simulink model "Differential_Jacobian_mapping_Model"  (R2016a)
settings: Solver=FixedStepAuto  SolverMode=SingleTasking  StartTime=0  StopTime=2  FixedStep=0.04  RelTol=1e-3
undefined symbols (not defined in the file): display, Z
libraries: sm_lib x176, nesl_utility x21, simulink x10
(part 2 of 2)

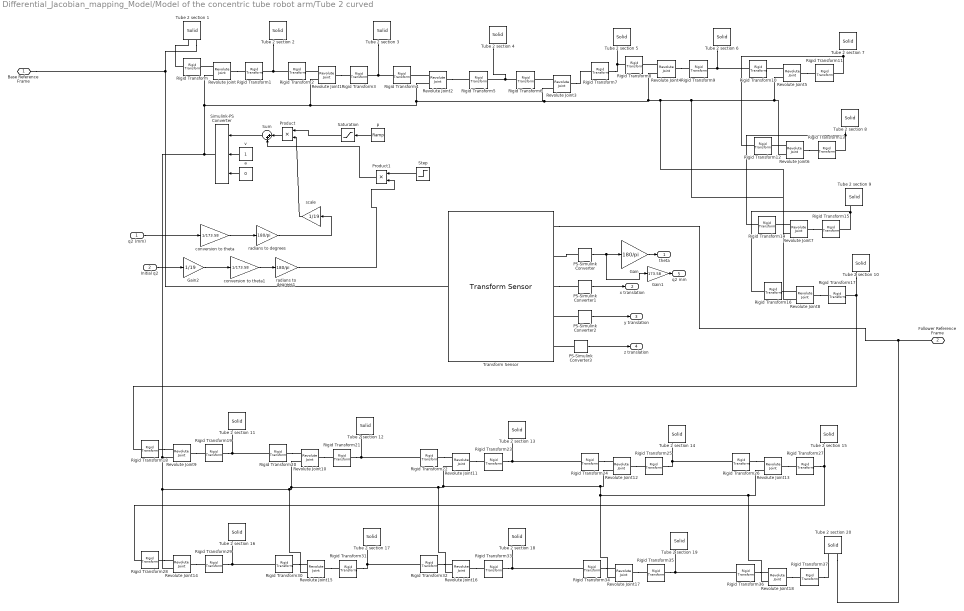
== system Differential_Jacobian_mapping_Model/Model of the concentric tube robot arm/Tube 2 curved ==
  q2 (mm) : Inport
  Initial q2 : Inport  Port=2
  Gain : Gain  Gain=180/pi
  Gain1 : Gain  Gain=173.58
  Gain2 : Gain  Gain=1/19
  PS-Simulink Converter{,1..3} (4 alike) : nesl_utility/PS-Simulink Converter  PhysicalDomain=network_engine_domain  SubClassName=ps_output  LeftPortType=input  RightPortType=output  PseudoPeriodic=off  Frequencies=[]  Unit=1  AffineConversion=off
  Product : Product
  Product1 : Product
  Revolute Joint{,1..18} (19 alike) : sm_lib/Joints/Revolute Joint  SenseConstraintForce=off  SenseConstraintForceX=off  SenseConstraintForceY=off  SenseConstraintForceZ=off  SenseConstraintTorque=off  SenseConstraintTorqueX=off  SenseConstraintTorqueY=off  SenseConstraintTorqueZ=off  SenseTotalForce=off  SenseTotalForceX=off  SenseTotalForceY=off  SenseTotalForceZ=off  SenseTotalTorque=off  SenseTotalTorqueX=off  SenseTotalTorqueY=off  SenseTotalTorqueZ=off  CompositeWrenchDir=FollowerOnBase  CompositeWrenchFrame=BaseFrame  EquilibriumPosition=0  EquilibriumPositionUnits=deg  SpringStiffness=0  SpringStiffnessUnits=N*m/deg  DampingCoefficient=0  DampingCoefficientUnits=N*m/(deg/s)  TorqueActuationMode=ComputedTorque  MotionActuationMode=InputMotion  SensePosition=off  SenseVelocity=off  SenseAcceleration=off  SenseTorqueForce=off  PositionTargetSpecify=off  PositionTargetPriority=High  PositionTargetValue=0  PositionTargetValueUnits=deg  VelocityTargetSpecify=off  VelocityTargetPriority=High  VelocityTargetValue=0  VelocityTargetValueUnits=deg/s
  Rigid Transform{,2,4,6,8,10,12,14,16,18,20,22,24,26,28,30,32,34,36} (19 alike) : sm_lib/Frames and Transforms/Rigid Transform  TranslationMethod=StandardAxis  TranslationLengthUnit=mm  TranslationStandardAxis=-X  TranslationStandardOffset=173.58  TranslationCartesianOffset=[0 0 0]  TranslationROffset=0  TranslationROffsetUnits=m  TranslationZOffset=0  TranslationZOffsetUnits=m  TranslationThetaOffset=0  TranslationThetaOffsetUnits=deg  RotationMethod=StandardAxis  RotationAngleUnits=deg  RotationStandardAxis=+X  RotationAngle=90  RotationArbitraryAxis=[0 0 1]  FollAlignAxisA=+X  BaseAlignAxisA=+Y  FollAlignAxisB=+Y  BaseAlignAxisB=+Z  RotationSequenceAxes=FollowerAxes  RotationSequence=XYX  RotationSequenceAngles=[0 0 0]  RotationSequenceAnglesUnits=deg  RotationMatrix=[1 0 0; 0 1 0; 0 0 1]
  Rigid Transform{1,3,5,7,9,11,13,15,17,19,21,23,25,27,29,31,33,35,37} (19 alike) : sm_lib/Frames and Transforms/Rigid Transform  TranslationMethod=StandardAxis  TranslationLengthUnit=mm  TranslationStandardAxis=+X  TranslationStandardOffset=173.58  TranslationCartesianOffset=[0 0 0]  TranslationROffset=0  TranslationROffsetUnits=m  TranslationZOffset=0  TranslationZOffsetUnits=m  TranslationThetaOffset=0  TranslationThetaOffsetUnits=deg  RotationMethod=StandardAxis  RotationAngleUnits=deg  RotationStandardAxis=-X  RotationAngle=90  RotationArbitraryAxis=[0 0 1]  FollAlignAxisA=+X  BaseAlignAxisA=+Y  FollAlignAxisB=+Y  BaseAlignAxisB=+Z  RotationSequenceAxes=FollowerAxes  RotationSequence=XYX  RotationSequenceAngles=[0 0 0]  RotationSequenceAnglesUnits=deg  RotationMatrix=[1 0 0; 0 1 0; 0 0 1]
  Saturation : Saturate  UpperLimit=1  LowerLimit=0
  Simulink-PS Converter : nesl_utility/Simulink-PS Converter  PhysicalDomain=network_engine_domain  SubClassName=ps_input  LeftPortType=input  RightPortType=output  PseudoPeriodic=off  Frequencies=[]  NoiseDistribution=none  NoiseParameters=[]  Unit=deg  AffineConversion=off  InputFiltering=derivs  SimscapeFilterOrder=1  InputFilterTimeConstant=0.001  UdotUserProvided=2
  Step : Step  Time=0  SampleTime=0
  Sum : Sum  Inputs=|++
  Transform Sensor : sm_lib/Frames and Transforms/Transform Sensor  MeasurementFrame=Base  SenseAngle=on  SenseAxis=off  SenseAngle1=off  SenseAngle2=off  SenseAngle3=off  SenseQ=off  SenseR=off  SenseOmegaX=off  SenseOmegaY=off  SenseOmegaZ=off  SenseOmega1=off  SenseOmega2=off  SenseOmega3=off  SenseQDot=off  SenseRDot=off  SenseAlphaX=off  SenseAlphaY=off  SenseAlphaZ=off  SenseAlpha1=off  SenseAlpha2=off  SenseAlpha3=off  SenseQDDot=off  SenseRDDot=off  SenseX=on  SenseY=on  SenseZ=on  SenseRad=off  SenseAzim=off  SenseDist=off  SenseInc=off  SenseXDot=off  SenseYDot=off  SenseZDot=off  SenseRadDot=off  SenseAzimDot=off  SenseDistDot=off  SenseIncDot=off  SenseXDDot=off  SenseYDDot=off  SenseZDDot=off  SenseRadDDot=off  SenseAzimDDot=off  SenseDistDDot=off  SenseIncDDot=off
  Tube 2 section {1..20} (20 alike) : sm_lib/Body Elements/Solid  InertiaType=CalculateFromGeometry  Mass=1  MassUnits=kg  CenterOfMass=[0 0 0]  CenterOfMassUnits=m  MomentsOfInertia=[1 1 1]  MomentsOfInertiaUnits=kg*m^2  ProductsOfInertia=[0 0 0]  ProductsOfInertiaUnits=kg*m^2  DensityBased=on  Density=1000  DensityUnits=kg/(m^3)  DoExposeReferenceFrame=on  SerializedFrames=<Frames><Frame><Id>Frame1</Id><Value><Name>F1</Name><Origin><Source>GeometricFeature</Source><FeatureName>back surface</FeatureName></Origin><PrimaryAxis><DefinedDirection>-Z</DefinedDirection><Source>GeometricFeature</Source><SourceDirection>+Z</SourceDirection><FeatureName>back surface</FeatureName></PrimaryAxis><SecondaryAxis><DefinedDirection>+X</DefinedDirection><Source>ReferenceFrame</Source><SourceDirection>+X</SourceDirection><FeatureName></FeatureName></SecondaryAxis></Value></Frame><Frame><Id>Frame2</Id><Value><Name>F2</Name><Origin><Source>GeometricFeature</Source><FeatureName>front surface</FeatureName></Origin><PrimaryAxis><DefinedDirection>+Z</DefinedDirection><Source>GeometricFeature</Source><SourceDirection>+Z</SourceDirection><FeatureName>front surface</FeatureName></PrimaryAxis><SecondaryAxis><DefinedDirection>+X</DefinedDirection><Source>ReferenceFrame</Source><SourceDirection>+X</SourceDirection><FeatureName></FeatureName></SecondaryAxis></Value></Frame></Frames>  GraphicType=FromGeometry  MarkerShape=Sphere  MarkerSize=10  GraphicVisPropType=SimpleVisualProperties  GraphicDiffuseColor=[0.5 0.5 0.5]  GraphicSpecularColor=[0.5 0.5 0.5 1.0]  GraphicAmbientColor=[0.15 0.15 0.15 1.0]  GraphicEmissiveColor=[0.0 0.0 0.0 1.0]  GraphicShininess=75  GraphicOpacity=1.0  GeometryShape=GeneralSolidOfRevolution  RectangleSize=[1 1]  RectangleSizeUnits=m  BrickDimensions=[1 1 1]  BrickDimensionUnits=m  CylinderRadius=3  CylinderRadiusUnits=mm  CylinderLength=q1  CylinderLengthUnits=mm  SphereRadius=1  SphereRadiusUnits=m  EllipsoidRadii=[1 1 1]  EllipsoidRadiiUnits=m  ExtrusionCrossSection=[1 1; -1 1; -1 -1; 1 -1]  ExtrusionCrossSectionUnits=m  ExtrusionLength=1  ExtrusionLengthUnits=m  PolygonNumSides=3  PolygonOuterRadius=1  PolygonOuterRadiusUnits=m  ExtGeomFileType=STEP  ExtGeomFileUnits=m  RevolutionCrossSection=Cross_section_tube2  RevolutionCrossSectionUnits=mm  RevolutionExtent=Custom  RevolutionAngle=5  RevolutionAngleUnits=deg
  a : Constant  Value=0
  conversion to theta : Gain  Gain=1/173.58
  conversion to theta1 : Gain  Gain=1/173.58
  p : simulink/Sources/Ramp  slope=1  start=0  X0=0
  radians to degrees : Gain  Gain=180/pi
  radians to degrees1 : Gain  Gain=180/pi
  scale : Gain  Gain=1/19
  v : Constant
  Base Reference Frame : PMIOPort  Port=1  Side=Left
  Follower Reference Frame : PMIOPort  Port=2  Side=Right
  theta : Outport
  x translation : Outport  Port=2
  y translation : Outport  Port=3
  z translation : Outport  Port=4
  q2 mm : Outport  Port=5
  wires:
  a/1 -> Simulink-PS Converter/3
  v/1 -> Simulink-PS Converter/2
  p/1 -> Saturation/1
  PS-Simulink Converter/1 -> Gain1/1, Gain/1
  Gain/1 -> theta/1
  Saturation/1 -> Product/1
  conversion to theta/1 -> radians to degrees/1
  PS-Simulink Converter1/1 -> x translation/1
  PS-Simulink Converter2/1 -> y translation/1
  PS-Simulink Converter3/1 -> z translation/1
  q2 (mm)/1 -> conversion to theta/1
  Product1/1 -> Sum/2
  Step/1 -> Product1/1
  radians to degrees1/1 -> Product1/2
  conversion to theta1/1 -> radians to degrees1/1
  radians to degrees/1 -> scale/1
  Initial q2/1 -> Gain2/1
  Gain2/1 -> conversion to theta1/1
  Gain1/1 -> q2 mm/1
  scale/1 -> Product/2
  Product/1 -> Sum/1
  Sum/1 -> Simulink-PS Converter/1
  connections:
  Rigid Transform/LConn1 -- Tube 2 section 1/LConn1
  Rigid Transform1/RConn1 -- Tube 2 section 2/LConn1 -- Rigid Transform2/LConn1
  Revolute Joint/LConn2 -- Revolute Joint8/LConn2 -- Revolute Joint7/LConn2 -- Revolute Joint6/LConn2 -- Revolute Joint5/LConn2 -- Revolute Joint4/LConn2 -- Revolute Joint3/LConn2 -- Revolute Joint2/LConn2 -- Revolute Joint1/LConn2 -- Revolute Joint18/LConn2 -- Revolute Joint13/LConn2 -- Revolute Joint17/LConn2 -- Revolute Joint12/LConn2 -- Revolute Joint11/LConn2 -- Revolute Joint16/LConn2 -- Revolute Joint10/LConn2 -- Revolute Joint15/LConn2 -- Revolute Joint14/LConn2 -- Revolute Joint9/LConn2 -- Simulink-PS Converter/RConn1
  Rigid Transform3/RConn1 -- Tube 2 section 3/LConn1 -- Rigid Transform4/LConn1
  Rigid Transform6/LConn1 -- Tube 2 section 4/LConn1 -- Rigid Transform5/RConn1
  Tube 2 section 5/LConn1 -- Rigid Transform7/RConn1 -- Rigid Transform8/LConn1
  Rigid Transform10/LConn1 -- Tube 2 section 6/LConn1 -- Rigid Transform9/RConn1
  Rigid Transform12/LConn1 -- Tube 2 section 7/LConn1 -- Rigid Transform11/RConn1
  Rigid Transform13/RConn1 -- Tube 2 section 8/LConn1 -- Rigid Transform14/LConn1
  Rigid Transform16/LConn1 -- Tube 2 section 9/LConn1 -- Rigid Transform15/RConn1
  Transform Sensor/RConn1 -- Tube 2 section 20/LConn2 -- Follower Reference Frame/RConn1
  Revolute Joint8/RConn1 -- Rigid Transform17/LConn1
  Revolute Joint1/RConn1 -- Rigid Transform3/LConn1
  Revolute Joint8/LConn1 -- Rigid Transform16/RConn1
  Revolute Joint2/LConn1 -- Rigid Transform4/RConn1
  Tube 2 section 10/LConn1 -- Rigid Transform18/LConn1 -- Rigid Transform17/RConn1
  Revolute Joint7/RConn1 -- Rigid Transform15/LConn1
  Revolute Joint7/LConn1 -- Rigid Transform14/RConn1
  Tube 2 section 1/LConn2 -- Base Reference Frame/RConn1 -- Transform Sensor/LConn1
  Revolute Joint3/RConn1 -- Rigid Transform7/LConn1
  PS-Simulink Converter/LConn1 -- Transform Sensor/RConn2
  Revolute Joint5/RConn1 -- Rigid Transform11/LConn1
  Revolute Joint4/RConn1 -- Rigid Transform9/LConn1
  Revolute Joint/RConn1 -- Rigid Transform1/LConn1
  Revolute Joint/LConn1 -- Rigid Transform/RConn1
  Revolute Joint1/LConn1 -- Rigid Transform2/RConn1
  Revolute Joint2/RConn1 -- Rigid Transform5/LConn1
  Revolute Joint3/LConn1 -- Rigid Transform6/RConn1
  Revolute Joint6/RConn1 -- Rigid Transform13/LConn1
  Revolute Joint4/LConn1 -- Rigid Transform8/RConn1
  Revolute Joint5/LConn1 -- Rigid Transform10/RConn1
  Revolute Joint6/LConn1 -- Rigid Transform12/RConn1
  PS-Simulink Converter3/LConn1 -- Transform Sensor/RConn5
  PS-Simulink Converter2/LConn1 -- Transform Sensor/RConn4
  Transform Sensor/RConn3 -- PS-Simulink Converter1/LConn1
  Rigid Transform18/RConn1 -- Revolute Joint9/LConn1
  Revolute Joint9/RConn1 -- Rigid Transform19/LConn1
  Rigid Transform19/RConn1 -- Rigid Transform20/LConn1 -- Tube 2 section 11/LConn1
  Rigid Transform20/RConn1 -- Revolute Joint10/LConn1
  Revolute Joint10/RConn1 -- Rigid Transform21/LConn1
  Rigid Transform21/RConn1 -- Tube 2 section 12/LConn1 -- Rigid Transform22/LConn1
  Rigid Transform22/RConn1 -- Revolute Joint11/LConn1
  Revolute Joint11/RConn1 -- Rigid Transform23/LConn1
  Rigid Transform23/RConn1 -- Rigid Transform24/LConn1 -- Tube 2 section 13/LConn1
  Rigid Transform24/RConn1 -- Revolute Joint12/LConn1
  Revolute Joint12/RConn1 -- Rigid Transform25/LConn1
  Rigid Transform25/RConn1 -- Rigid Transform26/LConn1 -- Tube 2 section 14/LConn1
  Rigid Transform26/RConn1 -- Revolute Joint13/LConn1
  Revolute Joint13/RConn1 -- Rigid Transform27/LConn1
  Rigid Transform27/RConn1 -- Rigid Transform28/LConn1 -- Tube 2 section 15/LConn1
  Rigid Transform28/RConn1 -- Revolute Joint14/LConn1
  Revolute Joint14/RConn1 -- Rigid Transform29/LConn1
  Rigid Transform29/RConn1 -- Rigid Transform30/LConn1 -- Tube 2 section 16/LConn1
  Rigid Transform30/RConn1 -- Revolute Joint15/LConn1
  Revolute Joint15/RConn1 -- Rigid Transform31/LConn1
  Rigid Transform31/RConn1 -- Rigid Transform32/LConn1 -- Tube 2 section 17/LConn1
  Rigid Transform32/RConn1 -- Revolute Joint16/LConn1
  Revolute Joint16/RConn1 -- Rigid Transform33/LConn1
  Rigid Transform33/RConn1 -- Rigid Transform34/LConn1 -- Tube 2 section 18/LConn1
  Rigid Transform34/RConn1 -- Revolute Joint17/LConn1
  Revolute Joint17/RConn1 -- Rigid Transform35/LConn1
  Rigid Transform35/RConn1 -- Rigid Transform36/LConn1 -- Tube 2 section 19/LConn1
  Rigid Transform36/RConn1 -- Revolute Joint18/LConn1
  Revolute Joint18/RConn1 -- Rigid Transform37/LConn1
  Rigid Transform37/RConn1 -- Tube 2 section 20/LConn1

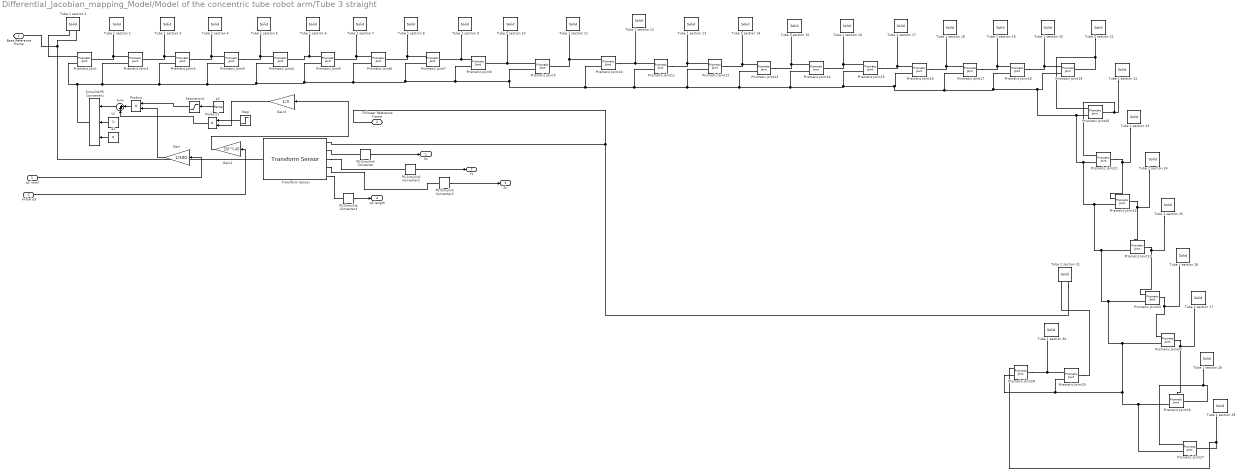
== system Differential_Jacobian_mapping_Model/Model of the concentric tube robot arm/Tube 3 straight ==
  q3 (mm) : Inport
  Initial q3 : Inport  Port=2
  Gain : Gain  Gain=1/300
  Gain2 : Gain  Gain=10^(-4)
  Gain3 : Gain  Gain=1/3
  PS-Simulink Converter{,1..3} (4 alike) : nesl_utility/PS-Simulink Converter  PhysicalDomain=network_engine_domain  SubClassName=ps_output  LeftPortType=input  RightPortType=output  PseudoPeriodic=off  Frequencies=[]  Unit=1  AffineConversion=off
  Prismatic Joint{,1..29} (30 alike) : sm_lib/Joints/Prismatic Joint  SenseConstraintForce=off  SenseConstraintForceX=off  SenseConstraintForceY=off  SenseConstraintForceZ=off  SenseConstraintTorque=off  SenseConstraintTorqueX=off  SenseConstraintTorqueY=off  SenseConstraintTorqueZ=off  SenseTotalForce=off  SenseTotalForceX=off  SenseTotalForceY=off  SenseTotalForceZ=off  SenseTotalTorque=off  SenseTotalTorqueX=off  SenseTotalTorqueY=off  SenseTotalTorqueZ=off  CompositeWrenchDir=FollowerOnBase  CompositeWrenchFrame=BaseFrame  EquilibriumPosition=0  EquilibriumPositionUnits=m  SpringStiffness=0  SpringStiffnessUnits=N/m  DampingCoefficient=0  DampingCoefficientUnits=N/(m/s)  TorqueActuationMode=ComputedTorque  MotionActuationMode=InputMotion  SensePosition=off  SenseVelocity=off  SenseAcceleration=off  SenseTorqueForce=off  PositionTargetSpecify=off  PositionTargetPriority=High  PositionTargetValue=0  PositionTargetValueUnits=m  VelocityTargetSpecify=off  VelocityTargetPriority=High  VelocityTargetValue=0  VelocityTargetValueUnits=m/s
  Product : Product
  Product1 : Product
  Saturation1 : Saturate  UpperLimit=0.01  LowerLimit=0
  Simulink-PS Converter1 : nesl_utility/Simulink-PS Converter  PhysicalDomain=network_engine_domain  SubClassName=ps_input  LeftPortType=input  RightPortType=output  PseudoPeriodic=off  Frequencies=[]  NoiseDistribution=none  NoiseParameters=[]  Unit=m  AffineConversion=off  InputFiltering=derivs  SimscapeFilterOrder=1  InputFilterTimeConstant=0.001  UdotUserProvided=2
  Step : Step  Time=0  SampleTime=0
  Sum : Sum  Inputs=|++
  Transform Sensor : sm_lib/Frames and Transforms/Transform Sensor  MeasurementFrame=Base  SenseAngle=off  SenseAxis=off  SenseAngle1=off  SenseAngle2=off  SenseAngle3=off  SenseQ=off  SenseR=off  SenseOmegaX=off  SenseOmegaY=off  SenseOmegaZ=off  SenseOmega1=off  SenseOmega2=off  SenseOmega3=off  SenseQDot=off  SenseRDot=off  SenseAlphaX=off  SenseAlphaY=off  SenseAlphaZ=off  SenseAlpha1=off  SenseAlpha2=off  SenseAlpha3=off  SenseQDDot=off  SenseRDDot=off  SenseX=on  SenseY=on  SenseZ=on  SenseRad=off  SenseAzim=off  SenseDist=on  SenseInc=off  SenseXDot=off  SenseYDot=off  SenseZDot=off  SenseRadDot=off  SenseAzimDot=off  SenseDistDot=off  SenseIncDot=off  SenseXDDot=off  SenseYDDot=off  SenseZDDot=off  SenseRadDDot=off  SenseAzimDDot=off  SenseDistDDot=off  SenseIncDDot=off
  Tube 1 section {1..31} (31 alike) : sm_lib/Body Elements/Solid  InertiaType=CalculateFromGeometry  Mass=1  MassUnits=kg  CenterOfMass=[0 0 0]  CenterOfMassUnits=m  MomentsOfInertia=[1 1 1]  MomentsOfInertiaUnits=kg*m^2  ProductsOfInertia=[0 0 0]  ProductsOfInertiaUnits=kg*m^2  DensityBased=on  Density=0  DensityUnits=kg/(m^3)  DoExposeReferenceFrame=on  SerializedFrames=<Frames><Frame><Id>Frame1</Id><Value><Name>F1</Name><Origin><Source>GeometricFeature</Source><FeatureName>bottom surface</FeatureName></Origin><PrimaryAxis><DefinedDirection>+Z</DefinedDirection><Source>ReferenceFrame</Source><SourceDirection>+Z</SourceDirection><FeatureName></FeatureName></PrimaryAxis><SecondaryAxis><DefinedDirection>+X</DefinedDirection><Source>ReferenceFrame</Source><SourceDirection>+X</SourceDirection><FeatureName></FeatureName></SecondaryAxis></Value></Frame><Frame><Id>Frame2</Id><Value><Name>F2</Name><Origin><Source>GeometricFeature</Source><FeatureName>top surface</FeatureName></Origin><PrimaryAxis><DefinedDirection>+Z</DefinedDirection><Source>ReferenceFrame</Source><SourceDirection>+Z</SourceDirection><FeatureName></FeatureName></PrimaryAxis><SecondaryAxis><DefinedDirection>+X</DefinedDirection><Source>ReferenceFrame</Source><SourceDirection>+X</SourceDirection><FeatureName></FeatureName></SecondaryAxis></Value></Frame></Frames>  GraphicType=FromGeometry  MarkerShape=Sphere  MarkerSize=10  GraphicVisPropType=SimpleVisualProperties  GraphicDiffuseColor=[0.5 0.5 0.5]  GraphicSpecularColor=[0.5 0.5 0.5 1.0]  GraphicAmbientColor=[0.15 0.15 0.15 1.0]  GraphicEmissiveColor=[0.0 0.0 0.0 1.0]  GraphicShininess=75  GraphicOpacity=1.0  GeometryShape=Cylinder  RectangleSize=[1 1]  RectangleSizeUnits=m  BrickDimensions=[1 1 1]  BrickDimensionUnits=m  CylinderRadius=0.5  CylinderRadiusUnits=mm  CylinderLength=10  CylinderLengthUnits=mm  SphereRadius=1  SphereRadiusUnits=m  EllipsoidRadii=[1 1 1]  EllipsoidRadiiUnits=m  ExtrusionCrossSection=[1 1; -1 1; -1 -1; 1 -1]  ExtrusionCrossSectionUnits=m  ExtrusionLength=1  ExtrusionLengthUnits=m  PolygonNumSides=3  PolygonOuterRadius=1  PolygonOuterRadiusUnits=m  ExtGeomFileType=STEP  ExtGeomFileUnits=m  RevolutionCrossSection=[1 1; 1 -1; 2 -1; 2 1]  RevolutionCrossSectionUnits=m  RevolutionExtent=Full  RevolutionAngle=180  RevolutionAngleUnits=deg
  a1 : Constant  Value=0
  p1 : simulink/Sources/Ramp  slope=0.01  start=0  X0=0
  v1 : Constant
  Base Reference Frame : PMIOPort  Port=1  Side=Left
  Follower Reference Frame : PMIOPort  Port=2  Side=Right
  Xc : Outport
  Yc : Outport  Port=2
  Zc : Outport  Port=3
  q3 length : Outport  Port=4
  wires:
  a1/1 -> Simulink-PS Converter1/3
  v1/1 -> Simulink-PS Converter1/2
  p1/1 -> Saturation1/1
  PS-Simulink Converter/1 -> Xc/1
  PS-Simulink Converter1/1 -> Yc/1
  PS-Simulink Converter2/1 -> Zc/1
  PS-Simulink Converter3/1 -> q3 length/1
  q3 (mm)/1 -> Gain/1
  Step/1 -> Product1/1
  Product1/1 -> Sum/2
  Initial q3/1 -> Gain2/1
  Gain2/1 -> Gain3/1
  Gain3/1 -> Product1/2
  Saturation1/1 -> Product/1
  Product/1 -> Sum/1
  Gain/1 -> Product/2
  Sum/1 -> Simulink-PS Converter1/1
  connections:
  Simulink-PS Converter1/RConn1 -- Prismatic Joint/LConn2 -- Prismatic Joint29/LConn2 -- Prismatic Joint28/LConn2 -- Prismatic Joint27/LConn2 -- Prismatic Joint26/LConn2 -- Prismatic Joint25/LConn2 -- Prismatic Joint24/LConn2 -- Prismatic Joint23/LConn2 -- Prismatic Joint22/LConn2 -- Prismatic Joint21/LConn2 -- Prismatic Joint20/LConn2 -- Prismatic Joint19/LConn2 -- Prismatic Joint18/LConn2 -- Prismatic Joint17/LConn2 -- Prismatic Joint16/LConn2 -- Prismatic Joint15/LConn2 -- Prismatic Joint14/LConn2 -- Prismatic Joint13/LConn2 -- Prismatic Joint12/LConn2 -- Prismatic Joint11/LConn2 -- Prismatic Joint10/LConn2 -- Prismatic Joint9/LConn2 -- Prismatic Joint8/LConn2 -- Prismatic Joint7/LConn2 -- Prismatic Joint6/LConn2 -- Prismatic Joint5/LConn2 -- Prismatic Joint4/LConn2 -- Prismatic Joint3/LConn2 -- Prismatic Joint2/LConn2 -- Prismatic Joint1/LConn2
  Tube 1 section 1/LConn1 -- Prismatic Joint/LConn1
  Prismatic Joint1/LConn1 -- Prismatic Joint/RConn1 -- Tube 1 section 2/LConn1
  Prismatic Joint2/LConn1 -- Prismatic Joint1/RConn1 -- Tube 1 section 3/LConn1
  Prismatic Joint3/LConn1 -- Tube 1 section 4/LConn1 -- Prismatic Joint2/RConn1
  Prismatic Joint4/LConn1 -- Tube 1 section 5/LConn1 -- Prismatic Joint3/RConn1
  Prismatic Joint4/RConn1 -- Tube 1 section 6/LConn1 -- Prismatic Joint5/LConn1
  Prismatic Joint6/LConn1 -- Prismatic Joint5/RConn1 -- Tube 1 section 7/LConn1
  Prismatic Joint7/LConn1 -- Prismatic Joint6/RConn1 -- Tube 1 section 8/LConn1
  Prismatic Joint8/LConn1 -- Prismatic Joint7/RConn1 -- Tube 1 section 9/LConn1
  Prismatic Joint9/LConn1 -- Tube 1 section 10/LConn1 -- Prismatic Joint8/RConn1
  Prismatic Joint9/RConn1 -- Prismatic Joint10/LConn1 -- Tube 1 section 11/LConn1
  Transform Sensor/LConn1 -- Base Reference Frame/RConn1 -- Tube 1 section 1/LConn2
  Follower Reference Frame/RConn1 -- Tube 1 section 31/LConn2 -- Transform Sensor/RConn1
  PS-Simulink Converter/LConn1 -- Transform Sensor/RConn2
  Transform Sensor/RConn3 -- PS-Simulink Converter1/LConn1
  Transform Sensor/RConn4 -- PS-Simulink Converter2/LConn1
  Prismatic Joint10/RConn1 -- Tube 1 section 12/LConn1 -- Prismatic Joint11/LConn1
  Prismatic Joint11/RConn1 -- Prismatic Joint12/LConn1 -- Tube 1 section 13/LConn1
  Prismatic Joint12/RConn1 -- Prismatic Joint13/LConn1 -- Tube 1 section 14/LConn1
  Prismatic Joint13/RConn1 -- Prismatic Joint14/LConn1 -- Tube 1 section 15/LConn1
  Prismatic Joint14/RConn1 -- Prismatic Joint15/LConn1 -- Tube 1 section 16/LConn1
  Prismatic Joint15/RConn1 -- Prismatic Joint16/LConn1 -- Tube 1 section 17/LConn1
  Prismatic Joint16/RConn1 -- Prismatic Joint17/LConn1 -- Tube 1 section 18/LConn1
  Prismatic Joint17/RConn1 -- Prismatic Joint18/LConn1 -- Tube 1 section 19/LConn1
  Prismatic Joint18/RConn1 -- Prismatic Joint19/LConn1 -- Tube 1 section 20/LConn1
  Tube 1 section 21/LConn1 -- Prismatic Joint20/LConn1 -- Prismatic Joint19/RConn1
  Tube 1 section 22/LConn1 -- Prismatic Joint21/LConn1 -- Prismatic Joint20/RConn1
  Prismatic Joint21/RConn1 -- Tube 1 section 23/LConn1 -- Prismatic Joint22/LConn1
  Prismatic Joint22/RConn1 -- Tube 1 section 24/LConn1 -- Prismatic Joint23/LConn1
  Prismatic Joint23/RConn1 -- Tube 1 section 25/LConn1 -- Prismatic Joint24/LConn1
  Prismatic Joint24/RConn1 -- Tube 1 section 26/LConn1 -- Prismatic Joint25/LConn1
  Prismatic Joint25/RConn1 -- Tube 1 section 27/LConn1 -- Prismatic Joint26/LConn1
  Prismatic Joint26/RConn1 -- Prismatic Joint27/LConn1 -- Tube 1 section 28/LConn1
  Tube 1 section 29/LConn1 -- Prismatic Joint28/LConn1 -- Prismatic Joint27/RConn1
  Prismatic Joint28/RConn1 -- Prismatic Joint29/LConn1 -- Tube 1 section 30/LConn1
  Prismatic Joint29/RConn1 -- Tube 1 section 31/LConn1
  Transform Sensor/RConn5 -- PS-Simulink Converter3/LConn1

== matlab function Differential_Jacobian_mapping_Model/Jacobian Inverse Kinematics Code/Differential_Inverse_Kinematics_Code ==
  data: dx input; dq1 output; dy input; dz input; dp input; dRoll input; dq2 output; dq3 output; dq4 output; dq5 output; dq6 output; dq7 output; dd input; q1_in input; q2_in input; q3_in input; q6_in input
function [dq1,dq2,dq3,dq4,dq5,dq6,dq7] = fcn(dx,dy,dz,dp,dRoll,dd,q1_in,q2_in,q3_in,q6_in)
%This Code is the algorithm to solve the inverse kinematics.
%There are 3 cases, This code will give motor commands that will satisfy position the
%most it can before saturation of tube elongation

%Special Functions
coder.extrinsic('clc')
coder.extrinsic('display')
clc

%Algorithm Constants:
r = 173.58; %curved pipe curvature
%Limits:
Qmin = [0 0 0 -4*pi]';
Qmax = [77.25 88.5 97.5 4*pi]';
Q6_offset = pi/2;
q6_in = q6_in - Q6_offset;

%Direct solution motors:
dq5 = 0; %Inactive motor
dq4 = dd;
dq7 = dRoll;

%RECALL INITIAL POSITION LOCATION:
%display('Start at X, Y, Z, P ');
X_in = (q3_in*sin(q2_in/r) + r*(1-cos(q2_in/r)))*cos(q6_in);
Y_in = (q3_in*sin(q2_in/r) + r*(1-cos(q2_in/r)))*sin(q6_in);
Z_in = q3_in*cos(q2_in/r) + r*sin(q2_in/r) + q1_in;
P_in = atan(sin(q6_in)*tan(q2_in/r));

%COMPUTE THE DESIRED END POSITION:
X_aim = X_in + dx;
Y_aim = Y_in + dy;
Z_aim = Z_in + dz;
P_aim = P_in + dp;

%initialise rate of change
dX = [0;0;0;0]; 
Q1_current = q1_in; Q2_current = q2_in; Q3_current = q3_in; Q6_current = q6_in; 

%Jacobian LOOP (in the actual snake robot this will be done in real time):

for i=1:80
    %Get current Position / orientation:
    %display('Currently at:');
X_current = (Q3_current*sin(Q2_current/r) + r*(1-cos(Q2_current/r)))*cos(Q6_current);
Y_current = (Q3_current*sin(Q2_current/r) + r*(1-cos(Q2_current/r)))*sin(Q6_current);
Z_current = Q3_current*cos(Q2_current/r) + r*sin(Q2_current/r) + Q1_current;
P_current = atan(sin(Q6_current)*tan(Q2_current/r));

%Substitute values into the Jacobian:
J = [ 0,                      cos(Q6_current)*(sin(Q2_current/r) + (Q3_current*cos(Q2_current/r))/r), sin(Q2_current/r)*cos(Q6_current),      sin(Q6_current)*(r*(cos(Q2_current/r) - 1) - Q3_current*sin(Q2_current/r))
      0,                      sin(Q6_current)*(sin(Q2_current/r) + (Q3_current*cos(Q2_current/r))/r), sin(Q2_current/r)*sin(Q6_current),     -cos(Q6_current)*(r*(cos(Q2_current/r) - 1) - Q3_current*sin(Q2_current/r))
      1,                                cos(Q2_current/r) - (Q3_current*sin(Q2_current/r))/r,         cos(Q2_current/r),                                               0
      0, (sin(Q6_current)*(tan(Q2_current/r)^2 + 1))/(r*(tan(Q2_current/r)^2*sin(Q6_current)^2 + 1)),                 0, (tan(Q2_current/r)*cos(Q6_current))/(tan(Q2_current/r)^2*sin(Q6_current)^2 + 1)];
    
  %Solve current rate of change aim:
dX(1) = X_aim - X_current; dX(2) = Y_aim - Y_current; dX(3) = Z_aim - Z_current; dX(4) = P_aim - P_current; 

    %Current motor values
    q = [Q1_current Q2_current Q3_current Q6_current];
    
  %Solve the Damping Least squares Matrix from Joint limit cost function
DL = eye(4); p = 2; c = 1; w = 1;
for j=1:4
    num = 2*q(j) - Qmax(j) - Qmin(j);
    den = Qmax(j) - Qmin(j);
    L = c*(num/den);
    DL(j,j) = L^p + w;  
end

   %Solve the motor rate of change: 
dQ = J' / (J*J' + DL) * dX;

    %Solve new current motor position
Q1_current = dQ(1) + Q1_current;
Q2_current = dQ(2) + Q2_current;
Q3_current = dQ(3) + Q3_current;
Q6_current = dQ(4) + Q6_current;

%Clip effect
if Q1_current > Qmax(1)
    Q1_current = Qmax(1);
elseif Q1_current < Qmin(1);
    Q1_current = Qmin(1);
end
if Q2_current > Qmax(2)
    Q2_current = Qmax(2);
elseif Q2_current < Qmin(2);
    Q2_current = Qmin(2);
end
if Q3_current > Qmax(3)
    Q3_current = Qmax(3);
elseif Q3_current < Qmin(3);
    Q3_current = Qmin(3);
end
    
end

%Grab final results
q1_final = Q1_current;
q2_final = Q2_current;
q3_final = Q3_current;
q6_final = Q6_current;

X_final = (q3_final*sin(q2_final/r) + r*(1-cos(q2_final/r)))*cos(q6_final);
Y_final = (q3_final*sin(q2_final/r) + r*(1-cos(q2_final/r)))*sin(q6_final);
Z_final = q3_final*cos(q2_final/r) + r*sin(q2_final/r) + q1_final;
P_final = atan(sin(q6_final)*tan(q2_final/r));

display('The given displacement is');
dX_given = X_final - X_in
dY_given = Y_final - Y_in 
dZ_given = Z_final - Z_in 
dP_given = P_final - P_in 
  
% OUTPUT THE CHANGE:
%display('The motor displacement is');
dq1 = q1_final - q1_in;
dq2 = q2_final - q2_in;
dq3 = q3_final - q3_in;
dq6 = q6_final - q6_in;

end
